simulink model "Design2"  (R2023b)
settings: Solver=FixedStepAuto  StartTime=0.0  StopTime=10.0  FixedStep=1e-3  RelTol=1e-3  EnableMultiTasking=on
undefined symbols (not defined in the file): D10, D11, D12, D13, D2, D4, D5, D7, D8, D9, PTA0, PTA2, PTB23, PTB9, PTC3, PTC4, PTD0, PTD1, PTD2, PTD3
libraries: frdmk64flib x10
settings Model: ExtModeTrigDuration=5  Creator=haley  LastModifiedBy=haley
settings OptimizationCC: EnhancedBackFolding=on  PassReuseOutputArgsAs=Individual arguments  ZeroExternalMemoryAtStartup=off  ZeroInternalMemoryAtStartup=off  MaxStackSize=64  OptimizeBlockOrder=speed  DifferentSizesBufferReuse=on  OptimizationCustomize=off  EfficientTunableParamExpr=on
settings DebuggingCC: ParameterTunabilityLossMsg=error
settings HardwareCC: ProdBitPerPointer=32  ProdBitPerSizeT=32  ProdBitPerPtrDiffT=32  ProdLargestAtomicInteger=Long  ProdLargestAtomicFloat=Double  ProdWordSize=32  ProdHWDeviceType=ARM Compatible->ARM Cortex
settings SFSimCC: MATLABDynamicMemAlloc=off
settings RTWCC: Description=Embedded Coder  SystemTargetFile=ert.tlc  HardwareBoard=NXP FRDM-K64F  TLCOptions="-aInlineSetEventsForThisBaseRateFcn=TLC_FALSE -aSuppressMultiTaskScheduler=TLC_FALSE  -aRateBasedStepFcn=0"  TemplateMakefile=ert_default_tmf  Toolchain=GNU Tools for ARM Embedded Processors
settings CodeAppCC: ForceParamTrailComments=on  IgnoreCustomStorageClasses=off  OperatorAnnotations=on  SimulinkDataObjDesc=on  SFDataObjDesc=on  InsertBlockDesc=on
settings ERTTargetCC: ExtModeTransport=4  ExtModeMexFile=sendToCommService

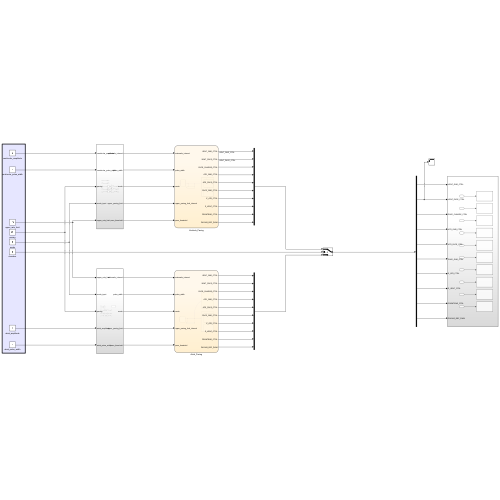
[thumbnail: Simulink's stored preview of the top-level diagram]
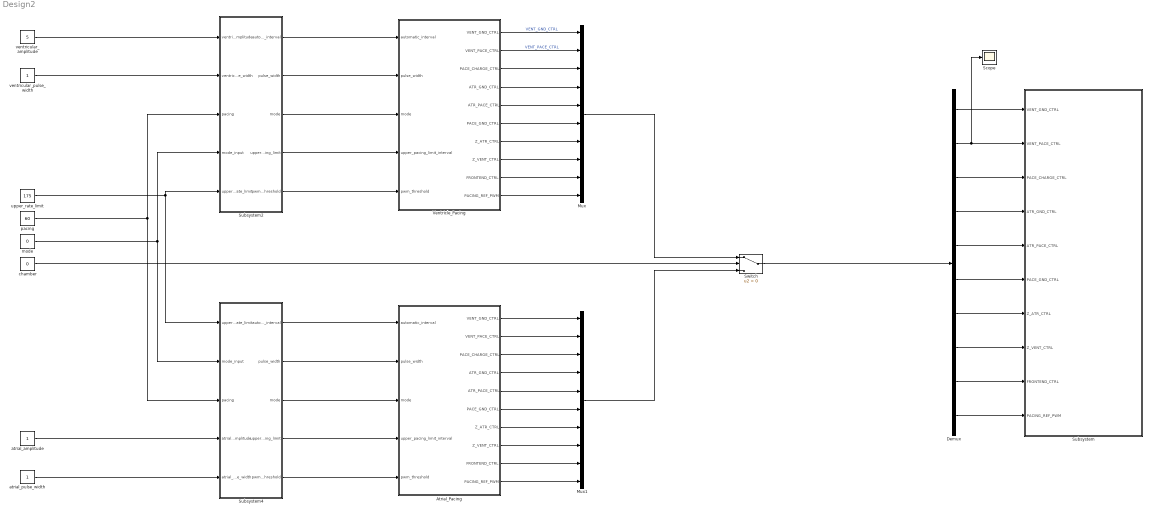
== system Design2 ==
  Atrial_Pacing : Stateflow chart  TreatAsAtomicUnit=on
      settings: PortSchema="{\"entries\":[{\"content\":{\"sides\":[{\"content\":{\"connectorIds\":[\"In1\",\"In2\",\"In3\",\"In4\",\"In5\"]},\"type\":\"ConnectorPlacement.EquallySpacedRectSide\",\"uuid\":\"0295b976-af9f-4ca7-b783-b7574ce7d878\"},{\"content\":{\"connectorIds\":[\"Out2\",\"Out3\",\"Out1\",\"Out8\",\"Out7\",\"Out4\",\"Out5\",\"Out6\",\"Out9\",\"Out10\"],\"side\":\"RIGHT\"},\"type\":\"ConnectorPlacement.EquallySpacedRectSide\",\"uuid\":\"8c797538-aae3-442d-b1de-b915081191d7\"},{\"content\":{\"side\":\"TOP\"},\"type\":\"ConnectorPlacement.EquallySpacedRectSide\",\"uuid\":\"af2b1efe-c74a-43e4-9bc2-de3c8cc2477c\"}]},\"type\":\"ConnectorPlacement.EquallySpacedConnector\",\"uuid\":\"3104347d-7f4e-4d45-9d00-2e2759d20ead\"}],\"packageUris\":[\"http://schema.mathworks.com/mf0/Connector/R2020b\"],\"version\":\"1.0\"}"
  Demux : Demux  Outputs=10
  Mux : Mux  Inputs=10
  Mux1 : Mux  Inputs=10
  Scope : Scope
  Subsystem : Subsystem
  Subsystem2 : Subsystem
  Subsystem4 : Subsystem
  Switch : Switch  Criteria=u2 > Threshold  SaturateOnIntegerOverflow=off  InputSameDT=off
  Ventricle_Pacing : Stateflow chart  TreatAsAtomicUnit=on
      settings: PortSchema="{\"entries\":[{\"content\":{\"sides\":[{\"content\":{\"connectorIds\":[\"In1\",\"In2\",\"In3\",\"In4\",\"In5\"]},\"type\":\"ConnectorPlacement.EquallySpacedRectSide\",\"uuid\":\"0295b976-af9f-4ca7-b783-b7574ce7d878\"},{\"content\":{\"connectorIds\":[\"Out2\",\"Out3\",\"Out1\",\"Out8\",\"Out7\",\"Out4\",\"Out5\",\"Out6\",\"Out9\",\"Out10\"],\"side\":\"RIGHT\"},\"type\":\"ConnectorPlacement.EquallySpacedRectSide\",\"uuid\":\"8c797538-aae3-442d-b1de-b915081191d7\"},{\"content\":{\"side\":\"TOP\"},\"type\":\"ConnectorPlacement.EquallySpacedRectSide\",\"uuid\":\"af2b1efe-c74a-43e4-9bc2-de3c8cc2477c\"}]},\"type\":\"ConnectorPlacement.EquallySpacedConnector\",\"uuid\":\"3104347d-7f4e-4d45-9d00-2e2759d20ead\"}],\"packageUris\":[\"http://schema.mathworks.com/mf0/Connector/R2020b\"],\"version\":\"1.0\"}"
  atrial_amplitude : Constant
  atrial_pulse_width : Constant
  chamber : Constant  Value=0
  mode : Constant  Value=0
  pacing : Constant  Value=60
  upper_rate_limit : Constant  Value=175
  ventricular_amplitude : Constant  Value=5
  ventricular_pulse_width : Constant
  wires:
  Subsystem2/1(automatic_interval) -> Ventricle_Pacing/1(automatic_interval)
  Subsystem2/2(pulse_width) -> Ventricle_Pacing/2(pulse_width)
  Ventricle_Pacing/2(VENT_GND_CTRL) -> Mux/1  "VENT_GND_CTRL"
  Ventricle_Pacing/3(VENT_PACE_CTRL) -> Mux/2  "VENT_PACE_CTRL"
  Ventricle_Pacing/1(PACE_CHARGE_CTRL) -> Mux/3
  Ventricle_Pacing/8(ATR_GND_CTRL) -> Mux/4
  Ventricle_Pacing/7(ATR_PACE_CTRL) -> Mux/5
  Ventricle_Pacing/4(PACE_GND_CTRL) -> Mux/6
  Ventricle_Pacing/5(Z_ATR_CTRL) -> Mux/7
  Ventricle_Pacing/6(Z_VENT_CTRL) -> Mux/8
  Ventricle_Pacing/9(FRONTEND_CTRL) -> Mux/9
  Mux/1 -> Switch/1
  Switch/1 -> Demux/1
  Demux/1 -> Subsystem/1(VENT_GND_CTRL)
  Demux/3 -> Subsystem/3(PACE_CHARGE_CTRL)
  Demux/4 -> Subsystem/4(ATR_GND_CTRL)
  Demux/5 -> Subsystem/5(ATR_PACE_CTRL)
  Demux/6 -> Subsystem/6(PACE_GND_CTRL)
  Demux/7 -> Subsystem/7(Z_ATR_CTRL)
  Demux/8 -> Subsystem/8(Z_VENT_CTRL)
  Demux/9 -> Subsystem/9(FRONTEND_CTRL)
  Subsystem2/3(mode) -> Ventricle_Pacing/3(mode)
  Atrial_Pacing/7(ATR_PACE_CTRL) -> Mux1/5
  Atrial_Pacing/4(PACE_GND_CTRL) -> Mux1/6
  Atrial_Pacing/8(ATR_GND_CTRL) -> Mux1/4
  Mux1/1 -> Switch/3
  Atrial_Pacing/1(PACE_CHARGE_CTRL) -> Mux1/3
  Atrial_Pacing/9(FRONTEND_CTRL) -> Mux1/9
  Atrial_Pacing/5(Z_ATR_CTRL) -> Mux1/7
  Atrial_Pacing/6(Z_VENT_CTRL) -> Mux1/8
  Subsystem4/1(automatic_interval) -> Atrial_Pacing/1(automatic_interval)
  Atrial_Pacing/3(VENT_PACE_CTRL) -> Mux1/2
  Subsystem4/2(pulse_width) -> Atrial_Pacing/2(pulse_width)
  Atrial_Pacing/2(VENT_GND_CTRL) -> Mux1/1
  Subsystem4/3(mode) -> Atrial_Pacing/3(mode)
  Subsystem2/4(upper_pacing_limit) -> Ventricle_Pacing/4(upper_pacing_limit_interval)
  Subsystem4/4(upper_pacing_limit) -> Atrial_Pacing/4(upper_pacing_limit_interval)
  Ventricle_Pacing/10(PACING_REF_PWM) -> Mux/10
  Atrial_Pacing/10(PACING_REF_PWM) -> Mux1/10
  Demux/10 -> Subsystem/10(PACING_REF_PWM)
  upper_rate_limit/1 -> Subsystem4/1(upper_rate_limit), Subsystem2/5(upper_rate_limit)
  mode/1 -> Subsystem4/2(mode_input), Subsystem2/4(mode_input)
  ventricular_amplitude/1 -> Subsystem2/1(ventricular_amplitude)
  ventricular_pulse_width/1 -> Subsystem2/2(ventricular_pulse_width)
  atrial_amplitude/1 -> Subsystem4/4(atrial_amplitude)
  atrial_pulse_width/1 -> Subsystem4/5(atrial_pulse_width)
  chamber/1 -> Switch/2
  Subsystem2/5(pwm_threshold) -> Ventricle_Pacing/5(pwm_threshold)
  Subsystem4/5(pwm_threshold) -> Atrial_Pacing/5(pwm_threshold)
  pacing/1 -> Subsystem2/3(pacing), Subsystem4/3(pacing)
  Demux/2 -> Subsystem/2(VENT_PACE_CTRL), Scope/1

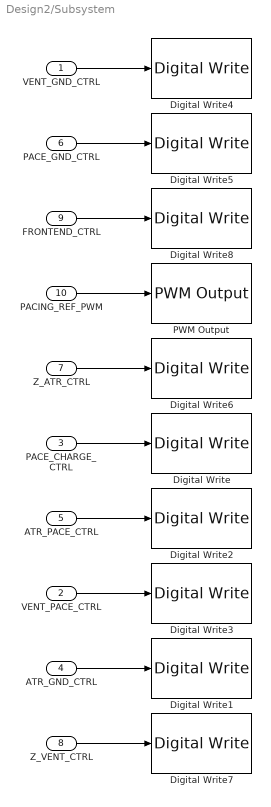
== system Design2/Subsystem ==
  VENT_GND_CTRL : Inport
  VENT_PACE_CTRL : Inport  Port=2
  PACE_CHARGE_CTRL : Inport  Port=3
  ATR_GND_CTRL : Inport  Port=4
  ATR_PACE_CTRL : Inport  Port=5
  PACE_GND_CTRL : Inport  Port=6
  Z_ATR_CTRL : Inport  Port=7
  Z_VENT_CTRL : Inport  Port=8
  FRONTEND_CTRL : Inport  Port=9
  PACING_REF_PWM : Inport  Port=10
  Digital Write : frdmk64flib/Digital Write  Whichpin=PTB9 (D2)
  Digital Write1 : frdmk64flib/Digital Write  Whichpin=PTD2 (D11)
  Digital Write2 : frdmk64flib/Digital Write  Whichpin=PTA0 (D8)
  Digital Write3 : frdmk64flib/Digital Write  Whichpin=PTC4 (D9)
  Digital Write4 : frdmk64flib/Digital Write  Whichpin=PTD3 (D12)
  Digital Write5 : frdmk64flib/Digital Write  Whichpin=PTD0 (D10)
  Digital Write6 : frdmk64flib/Digital Write  Whichpin=PTB23 (D4)
  Digital Write7 : frdmk64flib/Digital Write  Whichpin=PTC3 (D7)
  Digital Write8 : frdmk64flib/Digital Write  Whichpin=PTD1 (D13)
  PWM Output : frdmk64flib/PWM Output  Whichpin=PTA2 (D5)  InitialFrequency=2000  InitialDutyCycle=0
  wires:
  Z_ATR_CTRL/1 -> Digital Write6/1
  VENT_PACE_CTRL/1 -> Digital Write3/1
  FRONTEND_CTRL/1 -> Digital Write8/1
  PACING_REF_PWM/1 -> PWM Output/1
  ATR_PACE_CTRL/1 -> Digital Write2/1
  Z_VENT_CTRL/1 -> Digital Write7/1
  VENT_GND_CTRL/1 -> Digital Write4/1
  PACE_CHARGE_CTRL/1 -> Digital Write/1
  ATR_GND_CTRL/1 -> Digital Write1/1
  PACE_GND_CTRL/1 -> Digital Write5/1

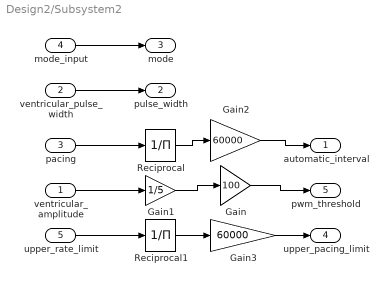
== system Design2/Subsystem2 ==
  ventricular_amplitude : Inport
  ventricular_pulse_width : Inport  Port=2
  pacing : Inport  Port=3
  mode_input : Inport  Port=4
  upper_rate_limit : Inport  Port=5
  Gain : Gain  Gain=100
  Gain1 : Gain  Gain=1/5
  Gain2 : Gain  Gain=60000
  Gain3 : Gain  Gain=60000
  Reciprocal : Product  Inputs=/
  Reciprocal1 : Product  Inputs=/
  automatic_interval : Outport
  pulse_width : Outport  Port=2
  mode : Outport  Port=3
  upper_pacing_limit : Outport  Port=4
  pwm_threshold : Outport  Port=5
  wires:
  mode_input/1 -> mode/1
  Gain1/1 -> Gain/1
  ventricular_amplitude/1 -> Gain1/1
  ventricular_pulse_width/1 -> pulse_width/1
  pacing/1 -> Reciprocal/1
  Reciprocal1/1 -> Gain3/1
  upper_rate_limit/1 -> Reciprocal1/1
  Reciprocal/1 -> Gain2/1
  Gain2/1 -> automatic_interval/1
  Gain/1 -> pwm_threshold/1
  Gain3/1 -> upper_pacing_limit/1

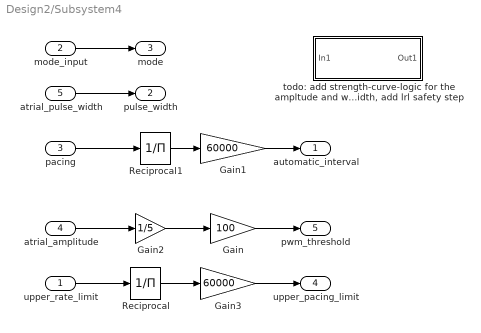
== system Design2/Subsystem4 ==
  upper_rate_limit : Inport
  mode_input : Inport  Port=2
  pacing : Inport  Port=3
  atrial_amplitude : Inport  Port=4
  atrial_pulse_width : Inport  Port=5
  Gain : Gain  Gain=100
  Gain1 : Gain  Gain=60000
  Gain2 : Gain  Gain=1/5
  Gain3 : Gain  Gain=60000
  Reciprocal : Product  Inputs=/
  Reciprocal1 : Product  Inputs=/
  "todo: add strength-curve-logic for the ampltude and width, add lrl safety step" : Subsystem
  automatic_interval : Outport
  pulse_width : Outport  Port=2
  mode : Outport  Port=3
  upper_pacing_limit : Outport  Port=4
  pwm_threshold : Outport  Port=5
  wires:
  atrial_amplitude/1 -> Gain2/1
  mode_input/1 -> mode/1
  atrial_pulse_width/1 -> pulse_width/1
  Gain2/1 -> Gain/1
  Gain1/1 -> automatic_interval/1
  Gain/1 -> pwm_threshold/1
  Gain3/1 -> upper_pacing_limit/1
  upper_rate_limit/1 -> Reciprocal/1
  Reciprocal/1 -> Gain3/1
  pacing/1 -> Reciprocal1/1
  Reciprocal1/1 -> Gain1/1

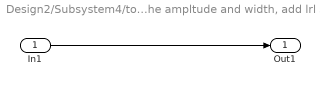
== system Design2/Subsystem4/todo: add strength-curve-logic for the ampltude and width, add lrl safety step ==
  In1 : Inport
  Out1 : Outport
  wires:
  In1/1 -> Out1/1

== stateflow chart Design2/Ventricle_Pacing ==
  state VOO
    state Charge_C22_Discharge_C21
      entry:
      %Charge C22
      VENT_PACE_CTRL = 0;
      PACE_CHARGE_CTRL = 1;
      %Discharge C21
      VENT_GND_CTRL= 1;
    state ChargeC21_and_DischargeC22
      %Creates the leading edge and sends pulse for X amount of time
      entry:
      PACE_CHARGE_CTRL = 0;
      VENT_GND_CTRL = 0;
      VENT_PACE_CTRL = 1;
      %Recharge pulse is the current in the opposite direction due to C21
    (default) -> Charge_C22_Discharge_C21
    Charge_C22_Discharge_C21 -> ChargeC21_and_DischargeC22 : after(c_automatic_interval-pulse_width, msec)
    ChargeC21_and_DischargeC22 -> Charge_C22_Discharge_C21 : after(pulse_width, msec)
  state Mode_Selection
    entry: %Safe State
    ATR_PACE_CTRL = 0;
    VENT_PACE_CTRL=0;
    PACING_REF_PWM = pwm_threshold;
    PACE_CHARGE_CTRL=0;
    PACE_GND_CTRL = 1;
    VENT_PACE_CTRL=0;
    Z_ATR_CTRL=0;
    Z_VENT_CTRL=0;
    ATR_PACE_CTRL=0;
    ATR_GND_CTRL=0;
    VENT_GND_CTRL=1;
    FRONTEND_CTRL=0;
    c_automatic_interval = automatic_interval;
  state SpeedGreaterThanUpperLimit
    entry:
    c_automatic_interval = upper_pacing_limit_interval
  (default) -> Mode_Selection
  Mode_Selection -> (junction 52)
  (junction 52) -> (junction 59) [order 2] : [automatic_interval<=upper_pacing_limit_interval]
  (junction 59) -> VOO : [mode==0]
  (junction 52) -> SpeedGreaterThanUpperLimit [order 1] : [automatic_interval>upper_pacing_limit_interval]
  SpeedGreaterThanUpperLimit -> (junction 59)
  data: automatic_interval input; pulse_width input; PACE_CHARGE_CTRL output; VENT_GND_CTRL output; VENT_PACE_CTRL output; mode input; PACE_GND_CTRL output; Z_ATR_CTRL output; Z_VENT_CTRL output; ATR_PACE_CTRL output; ATR_GND_CTRL output; FRONTEND_CTRL output; upper_pacing_limit_interval input; pwm_threshold input; PACING_REF_PWM output; c_automatic_interval local

== stateflow chart Design2/Atrial_Pacing ==
  state AAI
  state AOO
    state Charge_C22_Discharge_C21
      entry:
      %Charge C22
      ATR_PACE_CTRL = 0;
      PACE_CHARGE_CTRL = 1;
      %Discharge C21
      ATR_GND_CTRL= 1;
    state ChargeC21_and_DischargeC22
      %Creates the leading edge and sends pulse for X amount of time
      entry:
      PACE_CHARGE_CTRL = 0;
      ATR_PACE_CTRL = 1;
      ATR_GND_CTRL = 0;
    (default) -> Charge_C22_Discharge_C21
    Charge_C22_Discharge_C21 -> ChargeC21_and_DischargeC22 : after(c_automatic_interval-pulse_width, msec)
    ChargeC21_and_DischargeC22 -> Charge_C22_Discharge_C21 : after(pulse_width, msec)
  state Mode_Selection
    entry: %Safe State
    ATR_PACE_CTRL = 0;
    VENT_PACE_CTRL=0;
    PACING_REF_PWM = pwm_threshold;
    PACE_CHARGE_CTRL=0;
    PACE_GND_CTRL = 1;
    VENT_PACE_CTRL=0;
    Z_ATR_CTRL=0;
    Z_VENT_CTRL=0;
    ATR_PACE_CTRL=0;
    ATR_GND_CTRL=1;
    VENT_GND_CTRL=0;
    FRONTEND_CTRL=0;
    c_automatic_interval = automatic_interval;
  state SpeedGreaterThanUpperLimit
    entry:
    c_automatic_interval = upper_pacing_limit_interval
  (junction 52) -> AAI [order 2] : [mode == 1]
  Mode_Selection -> (junction 59)
  (junction 59) -> (junction 52) [order 2] : [automatic_interval<=upper_pacing_limit_interval]
  (junction 52) -> AOO [order 1] : [mode==0]
  (junction 59) -> SpeedGreaterThanUpperLimit [order 1] : [automatic_interval>upper_pacing_limit_interval]
  SpeedGreaterThanUpperLimit -> (junction 52)
  (default) -> Mode_Selection
  data: automatic_interval input; pulse_width input; PACE_CHARGE_CTRL output; VENT_GND_CTRL output; VENT_PACE_CTRL output; mode input; PACE_GND_CTRL output; Z_ATR_CTRL output; Z_VENT_CTRL output; ATR_PACE_CTRL output; ATR_GND_CTRL output; FRONTEND_CTRL output; upper_pacing_limit_interval input; PACING_REF_PWM output; pwm_threshold input; c_automatic_interval local
